simulink model "keypad_template"  (R2018b)
settings: Solver=ode1  StartTime=0.0  StopTime=inf  FixedStep=0.01  RelTol=1e-3  EnableMultiTasking=on
libraries: simulink x1
settings Model: SimulationMode=external  ExtModeTrigDuration=2  Creator=estra  LastModifiedBy=Ikarus
settings OptimizationCC: MaxStackSize=64
settings DebuggingCC: ParameterTunabilityLossMsg=error
settings HardwareCC: ProdBitPerInt=16  ProdBitPerPointer=16  ProdBitPerSizeT=16  ProdBitPerPtrDiffT=16  ProdLargestAtomicFloat=None  ProdWordSize=8  ProdHWDeviceType=Atmel->AVR
settings SFSimCC: SimUseLocalCustomCode=off  MATLABDynamicMemAlloc=off
settings RTWCC: SystemTargetFile=ert.tlc  HardwareBoard=Arduino Uno  TemplateMakefile=ert_default_tmf  GenerateReport=on  RTWUseLocalCustomCode=off  Toolchain=Arduino AVR  BuildConfiguration=Faster Runs  IncludeHyperlinkInReport=on  LaunchReport=on  GenerateTraceInfo=on  GenerateTraceReport=on  GenerateTraceReportSl=on  GenerateTraceReportSf=on  GenerateTraceReportEml=on
settings CodeAppCC: ForceParamTrailComments=on  IgnoreCustomStorageClasses=off  OperatorAnnotations=on  SimulinkDataObjDesc=on  SFDataObjDesc=on  MATLABFcnDesc=on  InsertBlockDesc=on  StateflowObjectComments=on  MATLABSourceComments=on
settings ERTTargetCC: MultiwordLength=2048  SupportContinuousTime=on  SupportVariableSizeSignals=on

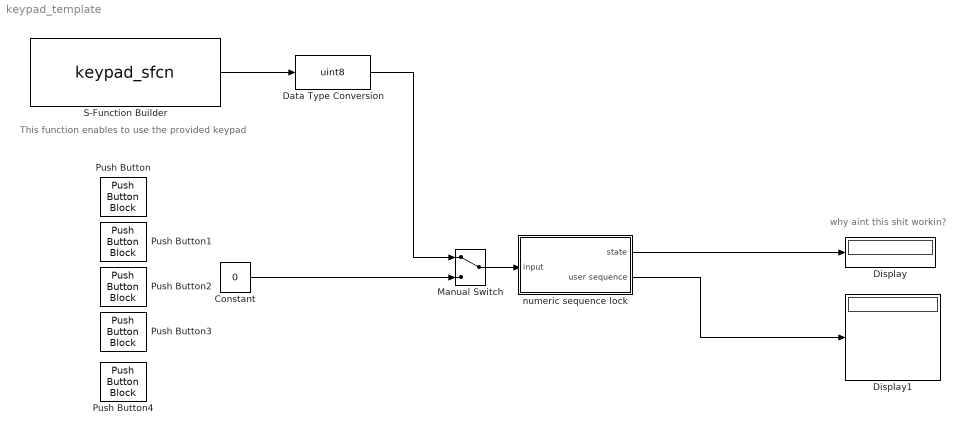
== system keypad_template ==
  note: why aint this shit workin?
  note: This function enables to use the provided keypad
  Constant : Constant  Value=0
  Data Type Conversion : DataTypeConversion  OutDataTypeStr=uint8
  Display : Display
  Display1 : Display
  Manual Switch : ManualSwitch
  Push Button : PushButtonBlock  WebBlockId=123  ButtonText=1  OnValue=49
  Push Button1 : PushButtonBlock  WebBlockId=124  ButtonText=2  OnValue=50
  Push Button2 : PushButtonBlock  WebBlockId=125  ButtonText=*  OnValue=42
  Push Button3 : PushButtonBlock  WebBlockId=126  ButtonText=#  OnValue=35
  Push Button4 : PushButtonBlock  WebBlockId=127  ButtonText=/  OnValue=47
  S-Function Builder : S-Function  InitFcn=try, set_param(gcb,'FunctionName','keypad_sfcn'), end  FunctionName=keypad_sfcn  SFunctionModules=keypad_sfcn_wrapper  SFunctionDeploymentMode=off  EnableBusSupport=off  mask(S-Function Builder){}
      mask help: Simulink:masks:SFunctionBuilder_MD
      mask init:
      | val = [[.9  0.75 0.75 1 1 .9 .9 1]',[1 1 0.75 0.75 .9 .9 1 .9]'];try , sys = get_param(gcb,'SfunBuilderFcnName');if isempty(sys), sys = get_param(gcb,'FunctionName'); end,catch, sys = get_param(gcb,'FunctionName'); end
      settings: CopyFcn=set_param(gcbh,'LinkStatus','none')  PreSaveFcn=try, set_param(gcb,'FunctionName','keypad_sfcn'), end  OpenFcn=sfunctionwizard(gcbh)
      mask Display: plot(val(:,1),val(:,2)),disp(sys), port_label('output',1,'y0')
  numeric sequence lock : Subsystem
  wires:
  S-Function Builder/1 -> Data Type Conversion/1
  numeric sequence lock/2(user sequence) -> Display1/1
  numeric sequence lock/1(state) -> Display/1
  Manual Switch/1 -> numeric sequence lock/1(input)
  Data Type Conversion/1 -> Manual Switch/1
  Constant/1 -> Manual Switch/2

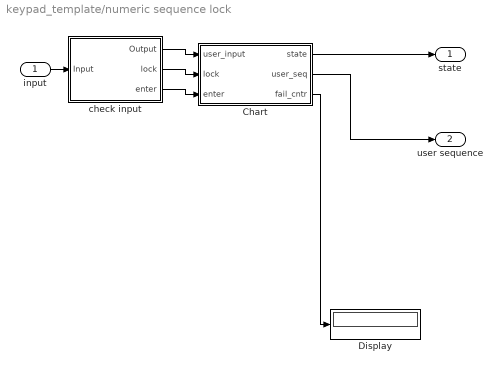
== system keypad_template/numeric sequence lock ==
  input : Inport
  Chart : Stateflow chart  TreatAsAtomicUnit=on
  Display : Display
  check input : Subsystem
  state : Outport
  user sequence : Outport  Port=2
  wires:
  check input/3(enter) -> Chart/3(enter)
  check input/2(lock) -> Chart/2(lock)
  check input/1("Output ") -> Chart/1(user_input)
  Chart/1(state) -> state/1
  Chart/2(user_seq) -> user sequence/1
  input/1 -> check input/1(Input)
  Chart/3(fail_cntr) -> Display/1

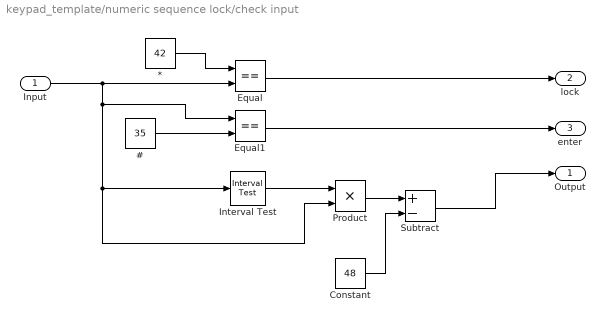
== system keypad_template/numeric sequence lock/check input ==
  Input : Inport
  # : Constant  Value=35
  * : Constant  Value=42
  Constant : Constant  Value=48
  Equal : RelationalOperator  Operator===  OutDataTypeStr=boolean  RndMeth=Simplest
  Equal1 : RelationalOperator  Operator===  OutDataTypeStr=boolean  RndMeth=Simplest
  "Interval Test " : simulink/Logic and Bit Operations/Interval Test  IntervalClosedRight=on  uplimit=57  IntervalClosedLeft=on  lowlimit=48  OutDataTypeStr=boolean
  Product : Product
  Subtract : Sum  Inputs=+-
  "Output " : Outport
  lock : Outport  Port=2
  enter : Outport  Port=3
  wires:
  */1 -> Equal/1
  Input/1 -> Product/2, "Interval Test "/1, Equal1/1, Equal/2
  #/1 -> Equal1/2
  "Interval Test "/1 -> Product/1
  Product/1 -> Subtract/1
  Constant/1 -> Subtract/2
  Subtract/1 -> "Output "/1
  Equal/1 -> lock/1
  Equal1/1 -> enter/1

== stateflow chart keypad_template/numeric sequence lock/Chart ==
  state INIT
    state = States.INIT
    sequence_length = 4
    fail_cntr = 0 %counts failed attemps
    seq_key = [1;1;1;1] %change this to change lock combination
  state LOCKED
    entry:
    state = States.LOCKED
    user_seq = [0;0;0;0] %resetting input
    i = 0 %reseting index
    %lock system
  state IDLE
    entry:
    state = States.IDLE
    %lock system
  state READING
    entry:
    state = States.READING
    i = i + 1 %increasing index
    user_seq(i) = user_input
  state CHECK
    entry:
    state = States.CHECK
  state UNLOCK
    entry:
    state = States.UNLOCK
    %do something
  state WRONG_CODE
    entry:
    state = States.WRONG_CODE
    fail_cntr = fail_cntr + 1
  state SYSTEM_LOCKDOWN
    entry:
    state = States.SYSTEM_LOCKDOWN
    %todo: implement delay
  (default) -> INIT
  UNLOCK -> INIT : [lock == 1]
  INIT -> LOCKED
  SYSTEM_LOCKDOWN -> LOCKED : [after(15,sec)]
  (junction 32) -> LOCKED [order 2]
  LOCKED -> IDLE
  (junction 42) -> IDLE [order 2] : [hasChanged(user_input)]
  IDLE -> READING : [hasChanged(user_input)]
  READING -> (junction 42)
  (junction 42) -> CHECK [order 1] : [i >= sequence_length]
  CHECK -> (junction 39) : [enter == 1]
  (junction 39) -> WRONG_CODE [order 2]
  (junction 39) -> UNLOCK [order 1] : [isequal(user_seq ,seq_key)]
  WRONG_CODE -> (junction 32)
  (junction 32) -> SYSTEM_LOCKDOWN [order 1] : [fail_cntr>=5]
  data: user_input input; state output Enum: States; i local; sequence_length local; seq_key local; sequece_length local; user_seq output size=4; lock input; enter input; fail_cntr output
